simulink library "INT_MeUn_Rot"  (R2016b)
settings: Solver=VariableStepAuto  StartTime=0.0  StopTime=10.0  RelTol=1e-3
settings Model: Creator=Administrator  LastModifiedBy=Administrator

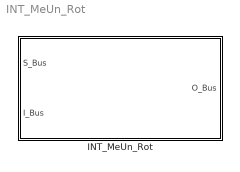
== system INT_MeUn_Rot ==
  INT_MeUn_Rot : Subsystem

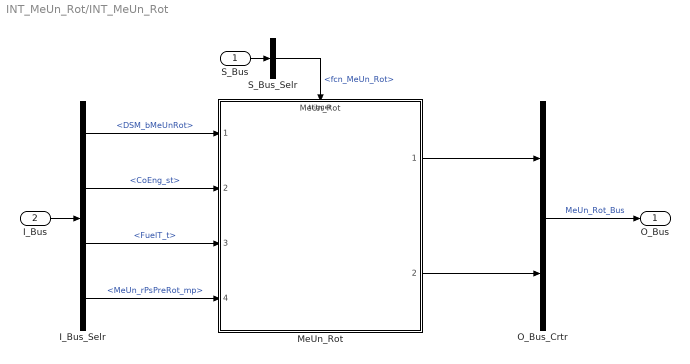
== system INT_MeUn_Rot/INT_MeUn_Rot ==
  S_Bus : Inport
  I_Bus : Inport  Port=2
  I_Bus_Selr : BusSelector  OutputSignals=DSM_bMeUnRot,CoEng_st,FuelT_t,MeUn_rPsPreRot_mp
  MeUn_Rot : ModelReference  ModelNameDialog=MeUn_Rot  SimulationMode=Normal  ModelReferenceVersion=1.4  TriggerPortName=function  TriggerPortTriggerType=function-call  TriggerPortStatesWhenEnabling=held
  O_Bus_Crtr : BusCreator  Inputs=2
  S_Bus_Selr : BusSelector  OutputSignals=fcn_MeUn_Rot
  O_Bus : Outport
  wires:
  S_Bus_Selr/1 -> MeUn_Rot/Trigger  "<fcn_MeUn_Rot>"
  S_Bus/1 -> S_Bus_Selr/1
  I_Bus/1 -> I_Bus_Selr/1
  I_Bus_Selr/1 -> MeUn_Rot/1  "<DSM_bMeUnRot>"
  I_Bus_Selr/2 -> MeUn_Rot/2  "<CoEng_st>"
  I_Bus_Selr/3 -> MeUn_Rot/3  "<FuelT_t>"
  I_Bus_Selr/4 -> MeUn_Rot/4  "<MeUn_rPsPreRot_mp>"
  O_Bus_Crtr/1 -> O_Bus/1  "MeUn_Rot_Bus"
  MeUn_Rot/1 -> O_Bus_Crtr/1
  MeUn_Rot/2 -> O_Bus_Crtr/2
